simulink model "lab_5"  (R2017a)
settings: Solver=FixedStepAuto  StartTime=0.0  StopTime=4.0  FixedStep=0.01  RelTol=1e-3
libraries: roblocks x3
settings Model: Creator=mkeari  LastModifiedBy=mkeari

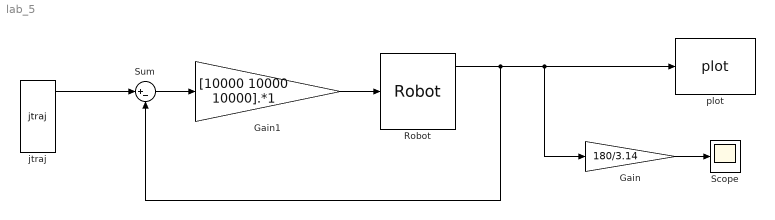
== system lab_5 ==
  Gain : Gain  Gain=180/3.14
  Gain1 : Gain  Gain=[10000 10000 10000].*1
  Robot : roblocks/Arm/Robot  robot=p560  q0=[0 0 0]
  Scope : Scope
  Sum : Sum  Inputs=|+-
  jtraj : roblocks/Toolbox/jtraj  q0=[0 0 0]  qf=[pi/2 -pi/4 -pi/4]  tmax=2  ts=0.02
  plot : roblocks/Arm/plot  robot=p560  fps=5  holdplot=on
  wires:
  Robot/1 -> Sum/2, Gain/1, plot/1
  Gain/1 -> Scope/1
  Sum/1 -> Gain1/1
  Gain1/1 -> Robot/1
  jtraj/1 -> Sum/1
